simulink model "actividad1_restore"  (R2021a)
settings: Solver=ode1  StartTime=0.0  StopTime=2  FixedStep=1e-5  RelTol=1e-3
libraries: pid_lib x1
settings Model: Creator=Agus  LastModifiedBy=zeta

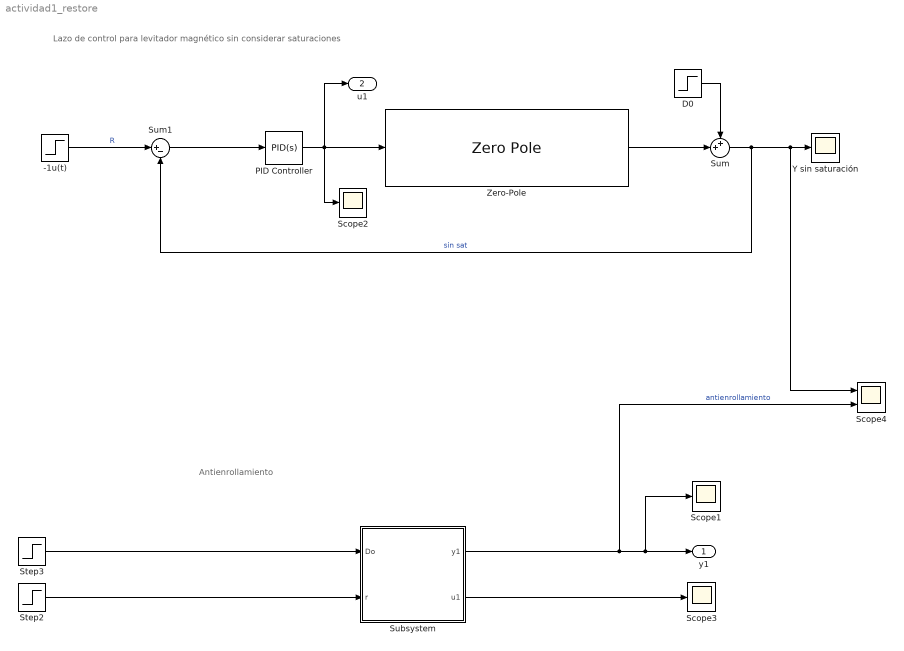
== system actividad1_restore ==
  note: Lazo de control para levitador magnético sin considerar saturaciones
  note: Antienrollamiento
  -1u(t) : Step  Time=0  After=-1  SampleTime=0
  D0 : Step  SampleTime=0
  PID Controller : pid_lib/PID Controller  Controller=PID  Form=Parallel  TimeDomain=Continuous-time  UseExternalTs=off  SampleTime=-1  IntegratorMethod=Forward Euler  FilterMethod=Forward Euler  ControllerParametersSource=internal  P=2.1595  I=8.175  D=0.0733  UseFilter=on  N=1364.25  TunerSelectOption=Transfer Function Based (PID Tuner App)  InitialConditionSource=internal  InitialConditionForIntegrator=0  InitialConditionForFilter=0  DifferentiatorICPrevScaledInput=0  ExternalReset=none  TrackingMode=off  Kt=1  LimitOutput=off  SatLimitsSource=internal  UpperSaturationLimit=inf  LowerSaturationLimit=-inf  LinearizeAsGain=on  AntiWindupMode=none  Kb=1  POutMin=[]  POutMax=[]  IOutMin=[]  IOutMax=[]  DOutMin=[]  DOutMax=[]  NOutMin=[]  NOutMax=[]  SumOutMin=[]  SumOutMax=[]  SaturationOutMin=[]  SaturationOutMax=[]  PParamMin=[]  PParamMax=[]  IParamMin=[]  IParamMax=[]  DParamMin=[]  DParamMax=[]  NParamMin=[]  NParamMax=[]  KbParamMin=[]  KbParamMax=[]  KtParamMin=[]  KtParamMax=[]  KbOutMin=[]  KbOutMax=[]  KtOutMin=[]  KtOutMax=[]  IntegratorOutMin=[]  IntegratorOutMax=[]  FilterOutMin=[]  FilterOutMax=[]  SumI1OutMin=[]  SumI1OutMax=[]  SumI2OutMin=[]  SumI2OutMax=[]  SumI3OutMin=[]  SumI3OutMax=[]  SumI4OutMin=[]  SumI4OutMax=[]  SumDOutMin=[]  SumDOutMax=[]  DifferentiatorOutMin=[]  DifferentiatorOutMax=[]  FilterDiffOutCoefMin=[]  FilterDiffOutCoefMax=[]  ReciprocalOutMin=[]  ReciprocalOutMax=[]  SumDenOutMin=[]  SumDenOutMax=[]  SumNumOutMin=[]  SumNumOutMax=[]  DivideOutMin=[]  DivideOutMax=[]  UdiffTsProdOutMin=[]  UdiffTsProdOutMax=[]  NTsProdOutMin=[]  NTsProdOutMax=[]  UintegralTsProdOutMin=[]  UintegralTsProdOutMax=[]  UngainTsProdOutMin=[]  UngainTsProdOutMax=[]  IntegratorContinuousStateAttributes=''  IntegratorStateMustResolveToSignalObject=off  IntegratorRTWStateStorageClass=Auto  FilterContinuousStateAttributes=''  FilterStateMustResolveToSignalObject=off  FilterRTWStateStorageClass=Auto  ParallelPVariant=InternalParameters  IdealPVariant=Disabled  IVariant=InternalParameters  DVariant=InternalParameters  IntegratorVariant=Continuous  SatVariant=Disabled  AWVariant=Passthrough  PCopyVariant=Disabled  TRVariant=Disabled  FdbkBlocksVariant=Forward  IdealPFdbkVariant=Disabled  SatFdbkVariant=Disabled  DerivativeFilterVariant=ContFilter  NVariant=InternalParameters  NCopyVariant=Disabled  FilterICVariant=InternalICsFilter  IntegratorICVariant=InternalICs  ExternalResetVariant=Disabled  TRSumVariant=Passthrough  SumFdbkVariant=Disabled  SumVariant=Sum_PID  TsampFilterVariant=InternalTs  TsampNgainVariant=Passthrough  TsampIntegralVariant=Passthrough  ExternalSaturationOutDataTypeStr=Inherit: Same as second input
  Scope1 : Scope
  Scope2 : Scope
  Scope3 : Scope
  Scope4 : Scope  NumInputPorts=2
  Step2 : Step  Time=0  After=-1  SampleTime=0
  Step3 : Step  SampleTime=0
  Subsystem : Subsystem  mask{Ki=8.175, Kp=2.1595, Kd=0.0733, tau=7.33e-4, sat=3.5}
  Sum : Sum  Inputs=++|
  Sum1 : Sum  Inputs=|+-
  Y sin saturación : Scope
  Zero-Pole : ZeroPole  Zeros=[]  Poles=[-100 -25 +25]  Gain=[57500]
  y1 : Outport
  u1 : Outport  Port=2
  wires:
  PID Controller/1 -> u1/1, Scope2/1, Zero-Pole/1
  Zero-Pole/1 -> Sum/2
  D0/1 -> Sum/1
  Sum1/1 -> PID Controller/1
  -1u(t)/1 -> Sum1/1  "R"
  Sum/1 -> Scope4/1, Y sin saturación/1, Sum1/2  "sin sat"
  Step3/1 -> Subsystem/1(Do)
  Step2/1 -> Subsystem/2(r)
  Subsystem/1(y1) -> Scope4/2, Scope1/1, y1/1  "antienrollamiento"
  Subsystem/2(u1) -> Scope3/1

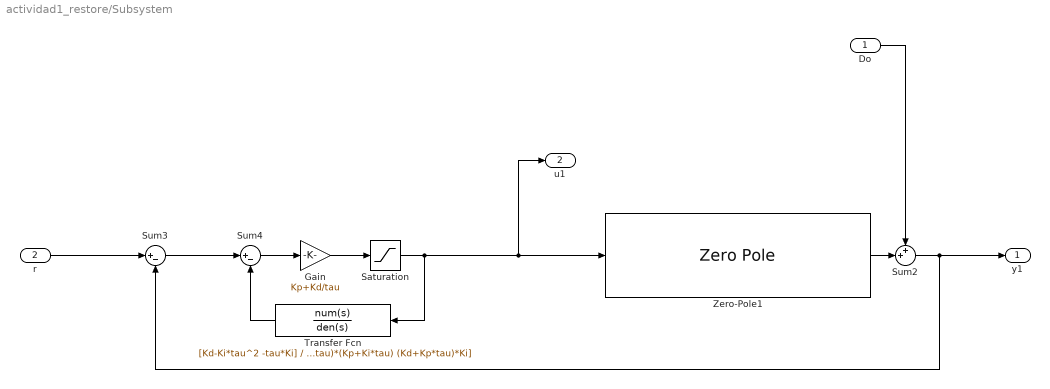
== system actividad1_restore/Subsystem ==
  Do : Inport
  r : Inport  Port=2
  Gain : Gain  Gain=Kp+Kd/tau
  Saturation : Saturate  UpperLimit=sat  LowerLimit=-sat
  Sum2 : Sum  Inputs=++|
  Sum3 : Sum  Inputs=|+-
  Sum4 : Sum  Inputs=|+-
  Transfer Fcn : TransferFcn  Numerator=[Kd-Ki*tau^2 -tau*Ki]  Denominator=[(Kd+Kp*tau)^2 (Kd+Kp*tau)*(Kp+Ki*tau) (Kd+Kp*tau)*Ki]
  Zero-Pole1 : ZeroPole  Zeros=[]  Poles=[-100 -25 +25]  Gain=[57500]
  y1 : Outport
  u1 : Outport  Port=2
  wires:
  Sum3/1 -> Sum4/1
  Zero-Pole1/1 -> Sum2/2
  Gain/1 -> Saturation/1
  Saturation/1 -> u1/1, Zero-Pole1/1, Transfer Fcn/1
  Sum2/1 -> y1/1, Sum3/2
  r/1 -> Sum3/1
  Transfer Fcn/1 -> Sum4/2
  Do/1 -> Sum2/1
  Sum4/1 -> Gain/1
